simulink library "csu_gpe_ground_point_extraction_lib"  (R2014b)
settings: Solver=ode45  SolverMode=SingleTasking  StartTime=0.0  StopTime=10.0  RelTol=1e-3
values from neighbouring files (symbols this model uses):
  cam_pixel_cols = 640    [csc_cam_camera_system_init.m]
  cam_pixel_rows = 480    [csc_cam_camera_system_init.m]
libraries: util_info_lib x1
settings Model: Creator=hcannon  LastModifiedBy=mstewart

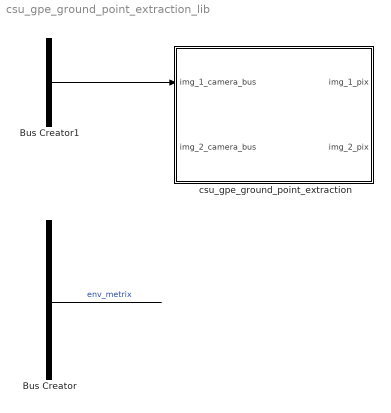
== system csu_gpe_ground_point_extraction_lib ==
  Bus Creator : BusCreator  Inputs=10
  Bus Creator1 : BusCreator  Inputs=5
  csu_gpe_ground_point_extraction : Subsystem
  wires:
  ? -> Bus Creator/10  "grv_gravity_acc_eci"
  ? -> Bus Creator/1  "rrd_alpha_body_in_eci"
  ? -> Bus Creator/2  "rrk_rate_body_eci_body"
  ? -> Bus Creator/3  "rrk_q_body_from_eci"
  ? -> Bus Creator/4  "rrk_euler_zyx_rot_deg"
  ? -> Bus Creator/5  "rtd_acc_body_in_eci"
  ? -> Bus Creator/6  "rtk_vel_eci"
  ? -> Bus Creator/7  "rtk_pos_eci"
  ? -> Bus Creator/8
  ? -> Bus Creator/9
  ? -> Bus Creator1/1  "cam_RW2C"
  ? -> Bus Creator1/4  "cam_projective_P"
  ? -> Bus Creator1/5  "cam_image_corners"
  ? -> Bus Creator1/2  "cam_position_T"
  ? -> Bus Creator1/3  "cam_Cext"
  Bus Creator1/1 -> csu_gpe_ground_point_extraction/1(img_1_camera_bus)
  Bus Creator/1 -> ?  "env_metrix"

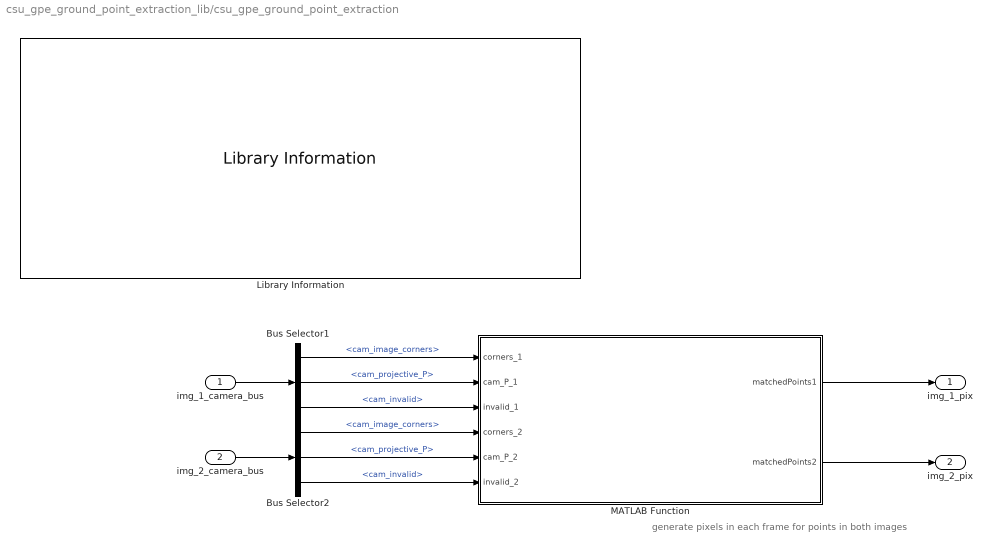
== system csu_gpe_ground_point_extraction_lib/csu_gpe_ground_point_extraction ==
  note: generate pixels in each frame for points in both images
  img_1_camera_bus : Inport
  img_2_camera_bus : Inport  Port=2
  Bus Selector1 : BusSelector  OutputSignals=cam_image_corners,cam_projective_P,cam_invalid
  Bus Selector2 : BusSelector  OutputSignals=cam_image_corners,cam_projective_P,cam_invalid
  Library Information : util_info_lib/Library Information  owner='NONE'
  MATLAB Function : MATLAB Function  TreatAsAtomicUnit=on
  img_1_pix : Outport
  img_2_pix : Outport  Port=2
  wires:
  Bus Selector2/3 -> MATLAB Function/6(invalid_2)  "<cam_invalid>"
  Bus Selector1/3 -> MATLAB Function/3(invalid_1)  "<cam_invalid>"
  Bus Selector1/1 -> MATLAB Function/1(corners_1)  "<cam_image_corners>"
  MATLAB Function/1(matchedPoints1) -> img_1_pix/1
  img_1_camera_bus/1 -> Bus Selector1/1
  Bus Selector1/2 -> MATLAB Function/2(cam_P_1)  "<cam_projective_P>"
  img_2_camera_bus/1 -> Bus Selector2/1
  Bus Selector2/1 -> MATLAB Function/4(corners_2)  "<cam_image_corners>"
  Bus Selector2/2 -> MATLAB Function/5(cam_P_2)  "<cam_projective_P>"
  MATLAB Function/2(matchedPoints2) -> img_2_pix/1

== matlab function csu_gpe_ground_point_extraction_lib/csu_gpe_ground_point_extraction/MATLAB Function ==
  data: corners_1 input double size=[4 3]; cam_P_1 input size=[3 4]; invalid_1 input; matchedPoints1 output double size=[16 2]; corners_2 input double size=[4 3]; cam_P_2 input double size=[3 4]; invalid_2 input; matchedPoints2 output double size=[16 2]; cam_pixel_rows parameter; cam_pixel_cols parameter
function [matchedPoints1,matchedPoints2] = ground_point_database(corners_1, cam_P_1,invalid_1, corners_2, cam_P_2, invalid_2, cam_pixel_rows, cam_pixel_cols)
%#codegen

npoints = 50;
range_x = max(corners_2(:,1)) - min(corners_2(:,1));
range_y = max(corners_2(:,2)) - min(corners_2(:,2));
xpoints = mean(corners_2(:,1)) + ( -range_x/2 + range_x*rand(npoints,1) );
ypoints = mean(corners_2(:,2)) + ( -range_y/2 + range_y*rand(npoints,1) );
zpoints = 0.01*abs((-5 + 20*rand(npoints,1)));

row1 = NaN(npoints,1);
col1 = NaN(npoints,1);
row2 = NaN(npoints,1);
col2 = NaN(npoints,1);
valid_match = zeros(npoints,1);
counter = 1;

for pp = 1 : length(xpoints)
    
    pix1 = cam_P_1*[xpoints(pp) ypoints(pp) zpoints(pp) 1]';
    pix1 = pix1(1:2)/pix1(3);
    
    pix2 = cam_P_2*[xpoints(pp) ypoints(pp) zpoints(pp) 1]';
    pix2 = pix2(1:2)/pix2(3);
    
    if ( pix1(1) > 0 && pix1(1) <= cam_pixel_cols) && ( pix1(2) > 0 && pix1(2) <= cam_pixel_rows)  && ( pix2(1) > 0 && pix2(1) <= cam_pixel_cols) && ( pix2(2) > 0 && pix2(2) <= cam_pixel_rows)
        
        row1(counter) = pix1(2);
        col1(counter) = pix1(1);
        
        row2(counter) = pix2(2);
        col2(counter) = pix2(1);
        
        valid_match(counter) = 1;

        counter = counter + 1;
        
    end
    
end

numToKeep = nnz(valid_match);

col1a = col1(1:16);
row1a = row1(1:16);
col2a = col2(1:16);
row2a = row2(1:16);

temp_matchedPoints1 = ([col1a row1a]);
temp_matchedPoints2 = ([col2a row2a]);

if invalid_1 > 0 || invalid_2 > 0
    numToKeep = 0;
end

matchedPoints1 = -1*ones(16,2);
matchedPoints2 = -1*ones(16,2);

n_matches = min(numToKeep,16);

for i = 1 : n_matches
    matchedPoints1(i,:) = temp_matchedPoints1(i,:);
    matchedPoints2(i,:) = temp_matchedPoints2(i,:);
end
